simulink model "TrackToTrackFusionSimulink"  (R2022a)
settings: Solver=FixedStepDiscrete  StartTime=0.0  StopTime=6.45  FixedStep=0.1  RelTol=1e-3
PreLoadFcn:
  | V1Sources(1).SourceIndex = 1;
  | V1Sources(1).IsInternalSource = true;
  | V1Sources(1).CentralToLocalTransformFcn = 'scenarioToEgo';
  | V1Sources(1).LocalToCentralTransformFcn = 'egoToScenario';
  | V1Sources(2).SourceIndex = 4;
  | V1Sources(2).IsInternalSource = false;
  | V1Sources(2).CentralToLocalTransformFcn = 'scenarioToEgo';
  | V1Sources(2).LocalToCentralTransformFcn = 'egoToScenario';
  | load('TrackToTrackFusionScenario.mat')
  | V2Sources(1).SourceIndex = 2;
  | V2Sources(1).IsInternalSource = true;
  | V2Sources(1).CentralToLocalTransformFcn = 'scenarioToEgo';
  | V2Sources(1).LocalToCentralTransformFcn = 'egoToScenario';
  | V2Sources(2).SourceIndex = 3;
  | V2Sources(2).IsInternalSource = false;
  | V2Sources(2).CentralToLocalTransformFcn = 'scenarioToEgo';
  | V2Sources(2).LocalToCentralTransformFcn = 'egoToScenario';
  | V3Sources(1).SourceIndex = 5;
  | V3Sources(1).IsInternalSource = true;
  | V3Sources(1).CentralToLocalTransformFcn = 'scenarioToEgo';
  | V3Sources(1).LocalToCentralTransformFcn = 'egoToScenario';
  | V3Sources(2).SourceIndex = 4;
  | V3Sources(2).IsInternalSource = false;
  | V3Sources(2).CentralToLocalTransformFcn = 'scenarioToEgo';
  | V3Sources(2).LocalToCentralTransformFcn = 'egoToScenario';
undefined symbols (not defined in the file or in its folder): driving, fusionCoordinateFrameType, matlabshared
libraries: drivingscenarioandsensors x7, motalgorithmslib x6, trackingutilitieslib x4
settings Model: Creator=The MathWorks, Inc.  LastModifiedBy=mciti
settings SolverCC: AlgebraicLoopSolver=TrustRegion  MaxZcPerStep=1
settings DebuggingCC: UnconnectedInputMsg=warning  UnconnectedOutputMsg=warning  UnconnectedLineMsg=warning  SFMachineParentedDataDiag=warning
settings RTWCC: DLArmComputeVersion=19.05

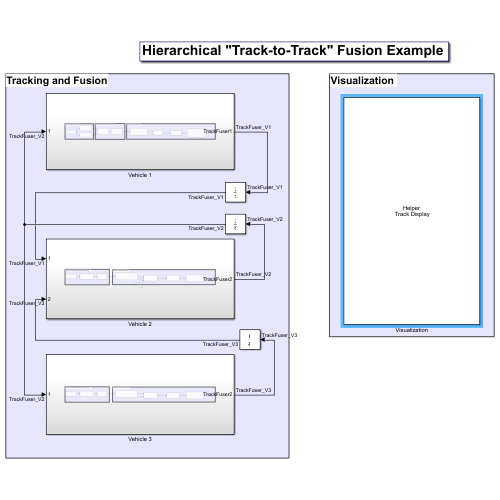
[thumbnail: Simulink's stored preview of the top-level diagram]
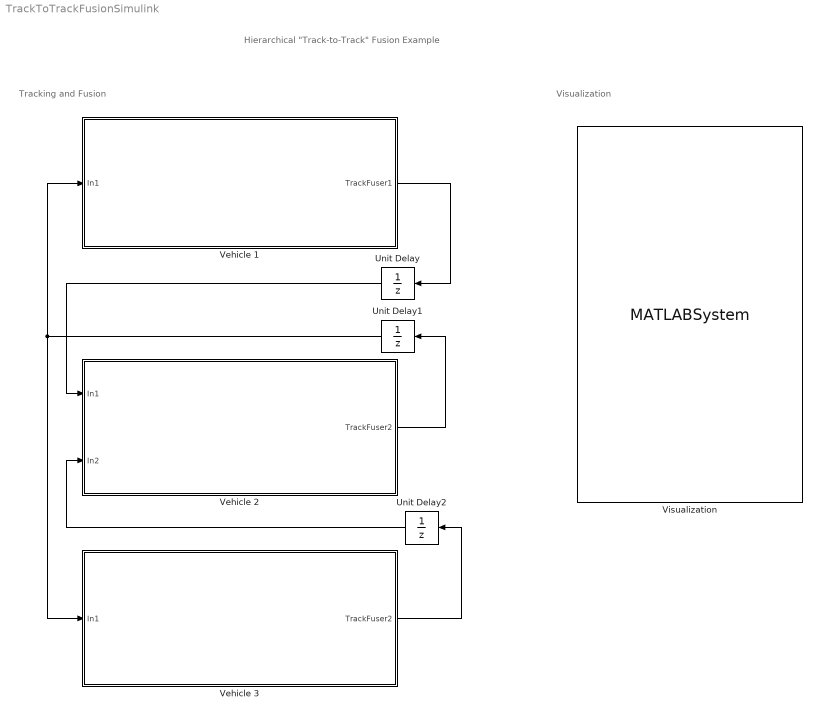
== system TrackToTrackFusionSimulink ==
  note: Tracking and Fusion
  note: Hierarchical "Track-to-Track" Fusion Example
  note: Visualization
  Unit Delay : UnitDelay  SampleTime=-1  StateName=TrackFuser_V1  HasFrameUpgradeWarning=on
  Unit Delay1 : UnitDelay  SampleTime=-1  StateName=TrackFuser_V2  HasFrameUpgradeWarning=on
  Unit Delay2 : UnitDelay  SampleTime=-1  StateName=TrackFuser_V2  HasFrameUpgradeWarning=on
  Vehicle 1 : Subsystem
  Vehicle 2 : Subsystem
  Vehicle 3 : Subsystem
  Visualization : MATLABSystem  System=HelperTrackDisplay  SubsystemBlockNames={ 'Vehicle 1', 'Vehicle 2' ,'Vehicle 3' }  PoseReaderBlockNames={ 'Detection Clustering', 'Detection Clustering' }  SourceTracksBlockNames={ 'JPDA Tracker V1', 'JPDA Tracker V2', 'JPDA Tracker V3' }  SourceUpdatePoseBlockNames={ 'Update Pose V1', 'Update Pose V2' ,'Update Pose V3' }  FusedTracksBlockNames={ 'T2TF Tracker V1', 'T2TF Tracker V2','T2TF Tracker V3' }  PosSelector=[ 1, 0, 0, 0, 0, 0; 0, 0, 1, 0, 0, 0; 0, 0, 0, 0, 1, 0 ]
      settings: ModelCloseFcn=helperCloseAll(gcb)
      mask Type: HelperTrackDisplay
      mask Display: disp(['Helper' char(10) ' Track Display']);
  wires:
  Unit Delay1/1 -> Vehicle 3/1(In1), Vehicle 1/1(In1)
  Vehicle 1/1(TrackFuser1) -> Unit Delay/1
  Unit Delay/1 -> Vehicle 2/1(In1)
  Vehicle 2/1(TrackFuser2) -> Unit Delay1/1
  Vehicle 3/1(TrackFuser2) -> Unit Delay2/1
  Unit Delay2/1 -> Vehicle 2/2(In2)

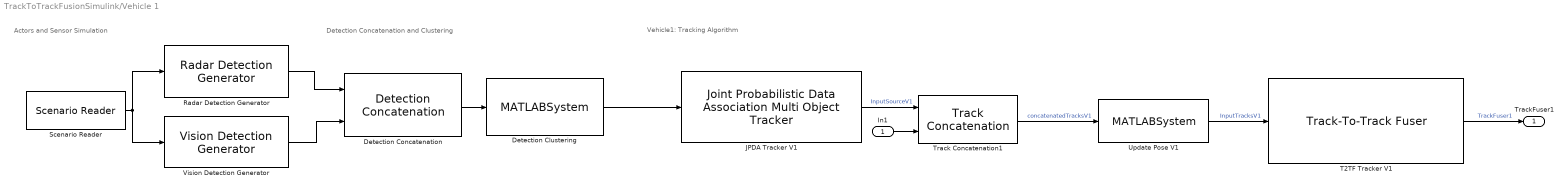
== system TrackToTrackFusionSimulink/Vehicle 1 ==
  note: Detection Concatenation and Clustering
  note: Vehicle1: Tracking Algorithm
  note: Actors and Sensor Simulation
  In1 : Inport
  Detection Clustering : MATLABSystem  System=helperClusterFuserDetections  ClusterSize=4.7  BusNameSource=Auto  BusName=BusClusterDetections  SimulateUsing=Code generation
      mask Type: helperClusterFuserDetections
      mask Display:
      | disp(['Detection' char(10) 'Clustering']);
      | port_label('input',1,'In');
      | port_label('output',1,'Out');
  Detection Concatenation : trackingutilitieslib/Detection Concatenation  NumInputs=2  BusNameSource=Auto  BusName=BusDetectionConcatenation  SimulateUsing=Interpreted execution
      settings: SourceProductBaseCode=TF,AE,DR,RA,UV,VE
  JPDA Tracker V1 : motalgorithmslib/Joint Probabilistic Data Association Multi Object Tracker  TrackerIndex=1  FilterInitializationFcn=initcvekf  MaxNumEvents=inf  EventGenerationFcn=jpdaEvents  MaxNumTracks=100  MaxNumSensors=2  TimeTolerance=1e-5  OOSMHandling=Terminate  MaxNumOOSMSteps=3  StateParametersSimulink=struct  HasStateParametersInput=off  EnableMemoryManagement=off  SimulateUsing=Interpreted execution  AssignmentThreshold=[ 1, Inf ] * 30  InitializationThreshold=0  DetectionProbability=0.9  ClutterDensity=1e-6  TrackLogic=History  pHistoryConfThreshold=[ 2, 3 ]  pHistoryDelThreshold=[ 3, 3 ]  pIntegratedConfThreshold=0.95  pIntegratedDelThreshold=0.1  HitMissThreshold=0.2  NewTargetDensity=1e-5  DeathRate=0.01  TimeInputSource=Auto  HasCostMatrixInput=off  HasDetectableTrackIDsInput=off  TentativeTracksOutputPort=off  AllTracksOutputPort=off  InfoOutputPort=off  BusNameSource=Auto  BusName=BusTrackerJPDA  BusName2Source=Auto  BusName2=BusTrackerInfo  MaxNumDetectionsPerSensor=100  MaxNumDetectionsPerCluster=5  MaxNumTracksPerCluster=5  ClusterViolationHandling=Split and warn
      settings: SourceProductBaseCode=TF
  Radar Detection Generator : drivingscenarioandsensors/Radar Detection Generator  SensorIndex=1  UpdateInterval=0.1  SensorLocation=[ 3.7, 0 ]  Height=0.2  Yaw=0  Pitch=0  Roll=0  BusNameSource=Auto  BusName=BusRadarDetectionGenerator  MaxNumDetectionsSource=Property  MaxNumDetections=50  DetectionCoordinates=Ego Cartesian  SimulateUsing=Interpreted execution  AzimuthResolution=4  ElevationResolution=10  RangeResolution=2.5  RangeRateResolution=0.5  AzimuthBiasFraction=0.1  ElevationBiasFraction=0.1  RangeBiasFraction=0.05  RangeRateBiasFraction=0.05  FieldOfView=[ 60, 5 ]  MaxRange=50  RangeRateLimits=[ -100, 100 ]  DetectionProbability=0.9  FalseAlarmRate=1e-6  ReferenceRange=100  ReferenceRCS=0  HasElevation=off  HasRangeRate=on  HasNoise=on  HasFalseAlarms=off  HasOcclusion=on  InitialSeedSource=Repeatable  InitialSeed=0  UsedSeed=matlabshared.tracking.internal.SimulinkUtilities.seedManager(gcb)  ActorProfilesSource=From Scenario Reader block  ActorProfilesParameters=driving.internal.ActorProfilesRadarParameters  ActorProfilesExpression=struct( 'ClassID', 0, 'Length', 4.7, 'Width', 1.8, 'Height', 1.4, 'OriginOffset', [ -1.35, 0, 0 ], 'RCSPattern', [ 10, 10; 10, 10 ], 'RCSAzimuthAngles', [ -180, 180 ], 'RCSElevationAngles', [ -90, 90 ] )
      settings: SourceProductBaseCode=DR
  Scenario Reader : drivingscenarioandsensors/Scenario Reader  ScenarioSource=From workspace  ScenarioFileName=EgoVehicleGoesStraight.mat  ScenarioVariableName=scenario  OutputCoordinateSystem=Vehicle coordinates  EgoVehicleSource=Scenario  EgoVehicleActorID=1  OrientVehiclesOnRoad=off  OutputEgoVehiclePose=off  OutputEgoVehicleState=off  SampleTime=0.1  LaneBoundaryOutput=None  LaneBoundaryDistance=0:0.5:9.5  LaneBoundaryLocation=Center of lane markings  BusNameSource=Auto  BusName=BusActors  BusNumActorsSource=Scenario  BusNumActors=100  BusName2Source=Auto  BusName2=BusLaneBoundaries  BusNumLaneBoundariesSource=Scenario  BusNumLaneBoundaries=10  BusName3Source=Auto  BusName3=BusEgoActor  BusName4Source=Auto  BusName4=BusEgoState  ShowCoordinateLabels=on  SimulateUsing=Interpreted execution
  T2TF Tracker V1 : motalgorithmslib/Track-To-Track Fuser  FuserIndex=3  Assignment=MatchPairs  AssignmentThreshold=[ 1, Inf ] * 30  MaxNumCentralTracks=100  MaxNumSources=2  SourceConfigurationExpression=V1Sources  IsSourceConfigurationsInput=off  StateParametersSimulink=struct('Frame',fusionCoordinateFrameType(1),'Position',[0 0 0],'Velocity',[0 0 0])  IsStateParametersInput=off  SimulateUsing=Interpreted execution  ConfirmationThreshold=[ 2, 3 ]  DeletionThreshold=[ 3, 3 ]  CentralTrackStateSize=6  CentralObjectAttributes=struct  StateTransitionFcn=constvel  ProcessNoise=eye( 3 )  HasAdditiveProcessNoise=off  StateFusion=Intersection  StateFusionParamSource=Auto  StateFusionCross=0.4  StateFusionIntersection=det  FuseConfirmedOnly=on  FuseCoasted=off  TimeInputSource=Auto  TentativeTracksOutputPort=off  AllTracksOutputPort=off  InfoOutputPort=off  BusNameSource=Property  BusName=TrackFuser_V1  BusName2Source=Auto  BusName2=BusTrackFuserInfo
      settings: SourceProductBaseCode=TF
  Track Concatenation1 : trackingutilitieslib/Track Concatenation  NumInputs=2  BusNameSource=Property  BusName=BusTrackConcatenation1  SimulateUsing=Interpreted execution
      settings: SourceProductBaseCode=TF,AE,DR,RA,UV,VE
  Update Pose V1 : MATLABSystem  System=HelperUpdatePose  DataFile={ 'v1Pose' }  DataVariableName=dataV1  TrackerId=1  BusNameSource=Property  BusName=UpdatePoseV1
      mask Type: HelperUpdatePose
      mask Display:
      | disp(['Helper' char(10) 'UpdatePose']);
      | port_label('input',1,'In');
      | port_label('output',1,'Tracks');
  Vision Detection Generator : drivingscenarioandsensors/Vision Detection Generator  SensorIndex=2  DetectorOutput=Objects only  UpdateInterval=0.1  LaneUpdateInterval=0.1  SensorLocation=[ 1.9, 0 ]  Height=1.1  Yaw=0  Pitch=1  Roll=0  BusNameSource=Auto  BusName=BusObjectDetections  BusName2Source=Auto  BusName2=BusLaneDetections  MaxNumDetectionsSource=Property  MaxNumDetections=50  MaxNumLanesSource=Property  MaxNumLanes=30  DetectionCoordinates=Ego Cartesian  SimulateUsing=Interpreted execution  MaxRange=100  BoundingBoxAccuracy=5  ProcessNoiseIntensity=5  MaxSpeed=100  MaxAllowedOcclusion=0.5  MinObjectImageSize=[ 15, 15 ]  DetectionProbability=0.9  FalsePositivesPerImage=0.1  MinLaneImageSize=[ 20, 3 ]  LaneBoundaryAccuracy=3  HasNoise=on  InitialSeedSource=Repeatable  InitialSeed=0  UsedSeed=driving.internal.SimulinkUtilities.seedManager(gcb)  ActorProfilesSource=From Scenario Reader block  ActorProfilesParameters=driving.internal.ActorProfilesParameters  ActorProfilesExpression=struct( 'ClassID', 0, 'Length', 4.7, 'Width', 1.8, 'Height', 1.4, 'OriginOffset', [ -1.35, 0, 0 ] )  Intrinsics=driving.internal.cameraIntrinsics
  TrackFuser1 : Outport
  wires:
  T2TF Tracker V1/1 -> TrackFuser1/1  "TrackFuser1"
  In1/1 -> Track Concatenation1/2
  JPDA Tracker V1/1 -> Track Concatenation1/1  "InputSourceV1"
  Track Concatenation1/1 -> Update Pose V1/1  "concatenatedTracksV1"
  Update Pose V1/1 -> T2TF Tracker V1/1  "InputTracksV1"
  Scenario Reader/1 -> Vision Detection Generator/1, Radar Detection Generator/1
  Radar Detection Generator/1 -> Detection Concatenation/1
  Vision Detection Generator/1 -> Detection Concatenation/2
  Detection Concatenation/1 -> Detection Clustering/1
  Detection Clustering/1 -> JPDA Tracker V1/1

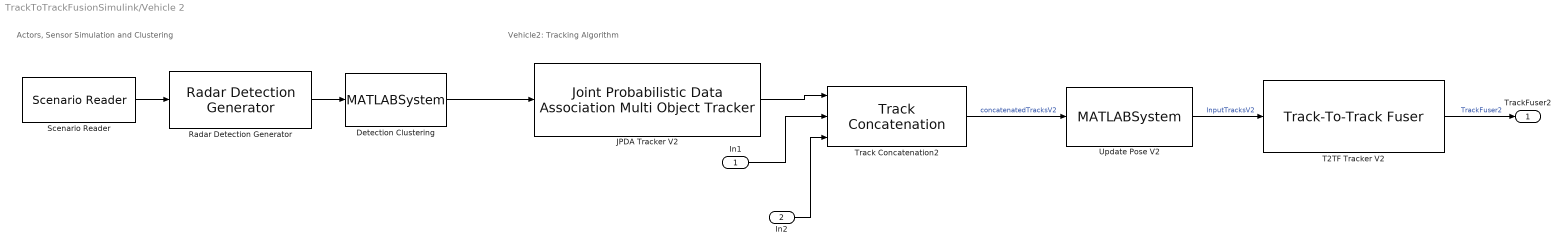
== system TrackToTrackFusionSimulink/Vehicle 2 ==
  note: Vehicle2: Tracking Algorithm
  note: Actors, Sensor Simulation and Clustering
  In1 : Inport
  In2 : Inport  Port=2
  Detection Clustering : MATLABSystem  System=helperClusterFuserDetections  ClusterSize=4.7  BusNameSource=Auto  BusName=BusClusterDetections  SimulateUsing=Code generation
      mask Type: helperClusterFuserDetections
      mask Display:
      | disp(['Detection' char(10) 'Clustering']);
      | port_label('input',1,'In');
      | port_label('output',1,'Out');
  JPDA Tracker V2 : motalgorithmslib/Joint Probabilistic Data Association Multi Object Tracker  TrackerIndex=2  FilterInitializationFcn=initcvekf  MaxNumEvents=inf  EventGenerationFcn=jpdaEvents  MaxNumTracks=100  MaxNumSensors=2  TimeTolerance=1e-5  OOSMHandling=Terminate  MaxNumOOSMSteps=3  StateParametersSimulink=struct  HasStateParametersInput=off  EnableMemoryManagement=off  SimulateUsing=Interpreted execution  AssignmentThreshold=[ 1, Inf ] * 30  InitializationThreshold=0  DetectionProbability=0.9  ClutterDensity=1e-6  TrackLogic=History  pHistoryConfThreshold=[ 2, 3 ]  pHistoryDelThreshold=[ 3, 3 ]  pIntegratedConfThreshold=0.95  pIntegratedDelThreshold=0.1  HitMissThreshold=0.2  NewTargetDensity=1e-5  DeathRate=0.01  TimeInputSource=Auto  HasCostMatrixInput=off  HasDetectableTrackIDsInput=off  TentativeTracksOutputPort=off  AllTracksOutputPort=off  InfoOutputPort=off  BusNameSource=Auto  BusName=BusTrackerJPDA  BusName2Source=Auto  BusName2=BusTrackerInfo  MaxNumDetectionsPerSensor=100  MaxNumDetectionsPerCluster=5  MaxNumTracksPerCluster=5  ClusterViolationHandling=Split and warn
      settings: SourceProductBaseCode=TF
  Radar Detection Generator : drivingscenarioandsensors/Radar Detection Generator  SensorIndex=3  UpdateInterval=0.1  SensorLocation=[ 3.7, 0 ]  Height=0.2  Yaw=0  Pitch=0  Roll=0  BusNameSource=Auto  BusName=BusRadarDetectionGenerator  MaxNumDetectionsSource=Property  MaxNumDetections=50  DetectionCoordinates=Ego Cartesian  SimulateUsing=Interpreted execution  AzimuthResolution=4  ElevationResolution=10  RangeResolution=2.5  RangeRateResolution=0.5  AzimuthBiasFraction=0.1  ElevationBiasFraction=0.1  RangeBiasFraction=0.05  RangeRateBiasFraction=0.05  FieldOfView=[ 30, 5 ]  MaxRange=120  RangeRateLimits=[ -100, 100 ]  DetectionProbability=0.9  FalseAlarmRate=1e-6  ReferenceRange=100  ReferenceRCS=0  HasElevation=off  HasRangeRate=on  HasNoise=on  HasFalseAlarms=off  HasOcclusion=on  InitialSeedSource=Repeatable  InitialSeed=0  UsedSeed=matlabshared.tracking.internal.SimulinkUtilities.seedManager(gcb)  ActorProfilesSource=From Scenario Reader block  ActorProfilesParameters=driving.internal.ActorProfilesRadarParameters  ActorProfilesExpression=struct( 'ClassID', 0, 'Length', 4.7, 'Width', 1.8, 'Height', 1.4, 'OriginOffset', [ -1.35, 0, 0 ], 'RCSPattern', [ 10, 10; 10, 10 ], 'RCSAzimuthAngles', [ -180, 180 ], 'RCSElevationAngles', [ -90, 90 ] )
      settings: SourceProductBaseCode=DR
  Scenario Reader : drivingscenarioandsensors/Scenario Reader  ScenarioSource=From workspace  ScenarioFileName=EgoVehicleGoesStraight.mat  ScenarioVariableName=scenario  OutputCoordinateSystem=Vehicle coordinates  EgoVehicleSource=Scenario  EgoVehicleActorID=2  OrientVehiclesOnRoad=off  OutputEgoVehiclePose=off  OutputEgoVehicleState=off  SampleTime=0.1  LaneBoundaryOutput=None  LaneBoundaryDistance=0:0.5:9.5  LaneBoundaryLocation=Center of lane markings  BusNameSource=Auto  BusName=BusActors  BusNumActorsSource=Scenario  BusNumActors=100  BusName2Source=Auto  BusName2=BusLaneBoundaries  BusNumLaneBoundariesSource=Scenario  BusNumLaneBoundaries=10  BusName3Source=Auto  BusName3=BusEgoActor  BusName4Source=Auto  BusName4=BusEgoState  ShowCoordinateLabels=on  SimulateUsing=Interpreted execution
  T2TF Tracker V2 : motalgorithmslib/Track-To-Track Fuser  FuserIndex=4  Assignment=MatchPairs  AssignmentThreshold=[ 1, Inf ] * 30  MaxNumCentralTracks=100  MaxNumSources=2  SourceConfigurationExpression=V2Sources  IsSourceConfigurationsInput=off  StateParametersSimulink=struct('Frame',fusionCoordinateFrameType(1),'Position',[0 0 0],'Velocity',[0 0 0])  IsStateParametersInput=off  SimulateUsing=Interpreted execution  ConfirmationThreshold=[ 2, 3 ]  DeletionThreshold=[ 3, 3 ]  CentralTrackStateSize=6  CentralObjectAttributes=struct  StateTransitionFcn=constvel  ProcessNoise=eye( 3 )  HasAdditiveProcessNoise=off  StateFusion=Intersection  StateFusionParamSource=Auto  StateFusionCross=0.4  StateFusionIntersection=det  FuseConfirmedOnly=on  FuseCoasted=off  TimeInputSource=Auto  TentativeTracksOutputPort=off  AllTracksOutputPort=off  InfoOutputPort=off  BusNameSource=Property  BusName=TrackFuser_V2  BusName2Source=Auto  BusName2=BusTrackFuserInfo
      settings: SourceProductBaseCode=TF
  Track Concatenation2 : trackingutilitieslib/Track Concatenation  NumInputs=3  BusNameSource=Property  BusName=TrackConcatenation2  SimulateUsing=Interpreted execution
      settings: SourceProductBaseCode=TF,AE,DR,RA,UV,VE
  Update Pose V2 : MATLABSystem  System=HelperUpdatePose  DataFile={ 'v2Pose' }  DataVariableName=dataV2  TrackerId=2  BusNameSource=Property  BusName=UpdatePoseV2
      mask Type: HelperUpdatePose
      mask Display:
      | disp(['Helper' char(10) 'UpdatePose']);
      | port_label('input',1,'In');
      | port_label('output',1,'Tracks');
  TrackFuser2 : Outport
  wires:
  T2TF Tracker V2/1 -> TrackFuser2/1  "TrackFuser2"
  In1/1 -> Track Concatenation2/2
  Update Pose V2/1 -> T2TF Tracker V2/1  "InputTracksV2"
  Track Concatenation2/1 -> Update Pose V2/1  "concatenatedTracksV2"
  Scenario Reader/1 -> Radar Detection Generator/1
  JPDA Tracker V2/1 -> Track Concatenation2/1
  Radar Detection Generator/1 -> Detection Clustering/1
  Detection Clustering/1 -> JPDA Tracker V2/1
  In2/1 -> Track Concatenation2/3

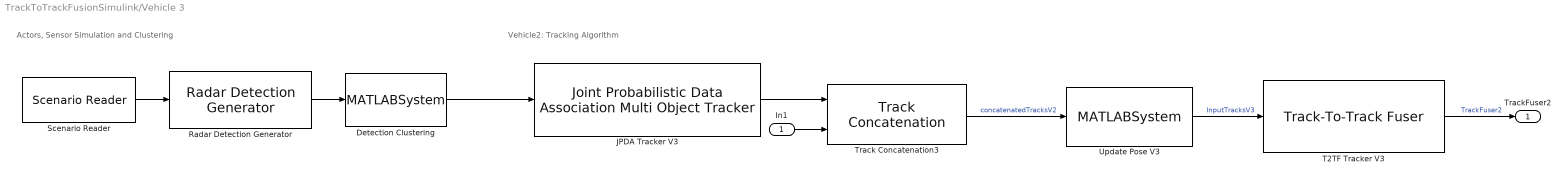
== system TrackToTrackFusionSimulink/Vehicle 3 ==
  note: Vehicle2: Tracking Algorithm
  note: Actors, Sensor Simulation and Clustering
  In1 : Inport
  Detection Clustering : MATLABSystem  System=helperClusterFuserDetections  ClusterSize=4.7  BusNameSource=Auto  BusName=BusClusterDetections  SimulateUsing=Code generation
      mask Type: helperClusterFuserDetections
      mask Display:
      | disp(['Detection' char(10) 'Clustering']);
      | port_label('input',1,'In');
      | port_label('output',1,'Out');
  JPDA Tracker V3 : motalgorithmslib/Joint Probabilistic Data Association Multi Object Tracker  TrackerIndex=5  FilterInitializationFcn=initcvekf  MaxNumEvents=inf  EventGenerationFcn=jpdaEvents  MaxNumTracks=100  MaxNumSensors=2  TimeTolerance=1e-5  OOSMHandling=Terminate  MaxNumOOSMSteps=3  StateParametersSimulink=struct  HasStateParametersInput=off  EnableMemoryManagement=off  SimulateUsing=Interpreted execution  AssignmentThreshold=[ 1, Inf ] * 30  InitializationThreshold=0  DetectionProbability=0.9  ClutterDensity=1e-6  TrackLogic=History  pHistoryConfThreshold=[ 2, 3 ]  pHistoryDelThreshold=[ 3, 3 ]  pIntegratedConfThreshold=0.95  pIntegratedDelThreshold=0.1  HitMissThreshold=0.2  NewTargetDensity=1e-5  DeathRate=0.01  TimeInputSource=Auto  HasCostMatrixInput=off  HasDetectableTrackIDsInput=off  TentativeTracksOutputPort=off  AllTracksOutputPort=off  InfoOutputPort=off  BusNameSource=Auto  BusName=BusTrackerJPDA  BusName2Source=Auto  BusName2=BusTrackerInfo  MaxNumDetectionsPerSensor=100  MaxNumDetectionsPerCluster=5  MaxNumTracksPerCluster=5  ClusterViolationHandling=Split and warn
      settings: SourceProductBaseCode=TF
  Radar Detection Generator : drivingscenarioandsensors/Radar Detection Generator  SensorIndex=6  UpdateInterval=0.1  SensorLocation=[ 3.7, 0 ]  Height=0.2  Yaw=0  Pitch=0  Roll=0  BusNameSource=Auto  BusName=BusRadarDetectionGenerator  MaxNumDetectionsSource=Property  MaxNumDetections=50  DetectionCoordinates=Ego Cartesian  SimulateUsing=Interpreted execution  AzimuthResolution=4  ElevationResolution=10  RangeResolution=2.5  RangeRateResolution=0.5  AzimuthBiasFraction=0.1  ElevationBiasFraction=0.1  RangeBiasFraction=0.05  RangeRateBiasFraction=0.05  FieldOfView=[ 30, 5 ]  MaxRange=120  RangeRateLimits=[ -100, 100 ]  DetectionProbability=0.9  FalseAlarmRate=1e-6  ReferenceRange=100  ReferenceRCS=0  HasElevation=off  HasRangeRate=on  HasNoise=on  HasFalseAlarms=off  HasOcclusion=on  InitialSeedSource=Repeatable  InitialSeed=0  UsedSeed=matlabshared.tracking.internal.SimulinkUtilities.seedManager(gcb)  ActorProfilesSource=From Scenario Reader block  ActorProfilesParameters=driving.internal.ActorProfilesRadarParameters  ActorProfilesExpression=struct( 'ClassID', 0, 'Length', 4.7, 'Width', 1.8, 'Height', 1.4, 'OriginOffset', [ -1.35, 0, 0 ], 'RCSPattern', [ 10, 10; 10, 10 ], 'RCSAzimuthAngles', [ -180, 180 ], 'RCSElevationAngles', [ -90, 90 ] )
      settings: SourceProductBaseCode=DR
  Scenario Reader : drivingscenarioandsensors/Scenario Reader  ScenarioSource=From workspace  ScenarioFileName=EgoVehicleGoesStraight.mat  ScenarioVariableName=scenario  OutputCoordinateSystem=Vehicle coordinates  EgoVehicleSource=Scenario  EgoVehicleActorID=3  OrientVehiclesOnRoad=off  OutputEgoVehiclePose=off  OutputEgoVehicleState=off  SampleTime=0.1  LaneBoundaryOutput=None  LaneBoundaryDistance=0:0.5:9.5  LaneBoundaryLocation=Center of lane markings  BusNameSource=Auto  BusName=BusActors  BusNumActorsSource=Scenario  BusNumActors=100  BusName2Source=Auto  BusName2=BusLaneBoundaries  BusNumLaneBoundariesSource=Scenario  BusNumLaneBoundaries=10  BusName3Source=Auto  BusName3=BusEgoActor  BusName4Source=Auto  BusName4=BusEgoState  ShowCoordinateLabels=on  SimulateUsing=Interpreted execution
  T2TF Tracker V3 : motalgorithmslib/Track-To-Track Fuser  FuserIndex=7  Assignment=MatchPairs  AssignmentThreshold=[ 1, Inf ] * 30  MaxNumCentralTracks=100  MaxNumSources=2  SourceConfigurationExpression=V3Sources  IsSourceConfigurationsInput=off  StateParametersSimulink=struct('Frame',fusionCoordinateFrameType(1),'Position',[0 0 0],'Velocity',[0 0 0])  IsStateParametersInput=off  SimulateUsing=Interpreted execution  ConfirmationThreshold=[ 2, 3 ]  DeletionThreshold=[ 3, 3 ]  CentralTrackStateSize=6  CentralObjectAttributes=struct  StateTransitionFcn=constvel  ProcessNoise=eye( 3 )  HasAdditiveProcessNoise=off  StateFusion=Intersection  StateFusionParamSource=Auto  StateFusionCross=0.4  StateFusionIntersection=det  FuseConfirmedOnly=on  FuseCoasted=off  TimeInputSource=Auto  TentativeTracksOutputPort=off  AllTracksOutputPort=off  InfoOutputPort=off  BusNameSource=Property  BusName=TrackFuser_V3  BusName2Source=Auto  BusName2=BusTrackFuserInfo
      settings: SourceProductBaseCode=TF
  Track Concatenation3 : trackingutilitieslib/Track Concatenation  NumInputs=2  BusNameSource=Property  BusName=TrackConcatenation3  SimulateUsing=Interpreted execution
      settings: SourceProductBaseCode=TF,AE,DR,RA,UV,VE
  Update Pose V3 : MATLABSystem  System=HelperUpdatePose  DataFile={ 'v3Pose' }  DataVariableName=dataV3  TrackerId=5  BusNameSource=Property  BusName=UpdatePoseV3
      mask Type: HelperUpdatePose
      mask Display:
      | disp(['Helper' char(10) 'UpdatePose']);
      | port_label('input',1,'In');
      | port_label('output',1,'Tracks');
  TrackFuser2 : Outport
  wires:
  T2TF Tracker V3/1 -> TrackFuser2/1  "TrackFuser2"
  In1/1 -> Track Concatenation3/2
  Update Pose V3/1 -> T2TF Tracker V3/1  "InputTracksV3"
  Track Concatenation3/1 -> Update Pose V3/1  "concatenatedTracksV2"
  Scenario Reader/1 -> Radar Detection Generator/1
  JPDA Tracker V3/1 -> Track Concatenation3/1
  Radar Detection Generator/1 -> Detection Clustering/1
  Detection Clustering/1 -> JPDA Tracker V3/1
